simulink model "Trajectory_tracking_full_state_feedback"  (R2023b)
settings: Solver=ode15s  StartTime=0.0  StopTime=tf+ss  FixedStep=Ts/10  MaxStep=Ts  RelTol=1e-12  AbsTol=1e-12
InitFcn:
  | %% Define the points of the curve
  | x=xp;
  | y=yp;
  | 
  | % Number of points
  | n = length(x);
  | 
  | % Initialize the arclength array
  | s = zeros(1, n);
  | 
  | %% Compute the incremental distances and the cumulative sum
  | for i = 2:n
  |     ds = sqrt((x(i) - x(i-1))^2 + (y(i) - y(i-1))^2);
  |     s(i) = s(i-1) + ds;
  | end
  | 
  | s= s/max(s);
  | 
  | [s, unique_indices] = unique(s, 'stable');
  | x = x(unique_indices);
  | y = y(unique_indices);
  | 
  | n = length(x);
  | 
  | %% Compute derivatives with respect to s
  | dx_ds = gradient(x, s);
  | dy_ds = gradient(y, s);
  | 
  | % Compute second derivatives with respect to s
  | d2x_ds2 = gradient(dx_ds, s);
  | d2y_ds2 = gradient(dy_ds, s);
  | 
  | % Compute third derivatives with respect to s
  | d3x_ds3 = gradient(d2x_ds2, s);
  | d3y_ds3 = gradient(d2y_ds2, s);
  | 
  | curvature = sqrt(d2x_ds2.^2+d2y_ds2.^2);
  | 
  | % % Dati Robot
  | CGTF=0.325;
  | CGTR=0.325;
  | Ts = 1/n;
  | 
  | 
  | %% Calcolo path
  | x_s= x;
  | y_s= y;
  | 
  | x_s_prime = dx_ds;
  | y_s_prime = dy_ds;
  | 
  | x_s_second = d2x_ds2;
  | y_s_second = d2y_ds2;
  | 
  | x_s_third = d3x_ds3;
  | y_s_third = d3y_ds3;
  | 
  | v_tilde = sqrt(x_s_prime.^2 + y_s_prime.^2);
  | 
  | theta_s = atan2(y_s_prime./v_tilde,x_s_prime./v_tilde);
  | theta_s_prime = (y_s_second.*x_s_prime-x_s_second.*y_s_prime)./(v_tilde.^2);
  | 
  | phi_s = atan(l*(y_s_second.*x_s_prime-x_s_second.*y_s_prime)./(v_tilde.^3));
  | 
  | w_tilde = (l*v_tilde.*((y_s_third.*x_s_prime-x_s_third.*y_s_prime)-3*(y_s_second.*x_s_prime-x_s_second.*y_s_prime).*(x_s_prime.*x_s_second+y_s_prime.*y_s_second)))./((v_tilde.^6)+(l^2)*(y_s_second.*x_s_prime-x_s_second.*y_s_prime).^2);
  | 
  | %% Time law
  | check=0;
  | t0 = 0;
  | tf = 1;
  | K=1;
  | while (~check)
  | 
  |     a0 = s(:,1);
  |     a1 = 0;
  |     a2 = 3/(tf^2)*(s(:,n)-s(:,1));
  |     a3 = -2/(tf^3)*(s(:,n)-s(:,1));
  | 
  |     % % Define the boundary conditions for s(t)
  |     % t0 = 0; % initial time
  |     % t_end = tf; % end time
  |     % s0 = s(:,1); % initial arc length
  |     % s_end = s(:,n); % end arc length
  |     % v0 = 0; % initial velocity
  |     % v_end = 0; % end velocity
  |     % a0 = 0; % initial acceleration
  |     % a_end = 0; % end acceleration
  |     %
  |     % % Set up the system of equations for quintic polynomial
  |     % A = [
  |     %     1, t0, t0^2, t0^3, t0^4, t0^5;
  |     %     1, t_end, t_end^2, t_end^3, t_end^4, t_end^5;
  |     %     0, 1, 2*t0, 3*t0^2, 4*t0^3, 5*t0^4;
  |     %     0, 1, 2*t_end, 3*t_end^2, 4*t_end^3, 5*t_end^4;
  |     %     0, 0, 2, 6*t0, 12*t0^2, 20*t0^3;
  |     %     0, 0, 2, 6*t_end, 12*t_end^2, 20*t_end^3
  |     % ];
  |     %
  |     % b = [s0; s_end; v0; v_end; a0; a_end];
  |     %
  |     % % Solve for the coefficients
  |     % coefficients = A\b;
  |     %
  |     % % Extract the coefficients
  |     % a0 = coefficients(1);
  |     % a1 = coefficients(2);
  |     % a2 = coefficients(3);
  |     % a3 = coefficients(4);
  |     % a4 = coefficients(5);
  |     % a5 = coefficients(6);
  | 
  |     % Define the quintic polynomial function s(t)
  |     % s_t = @(t) a0 + a1*t + a2*t^2 + a3*t^3 + a4*t^4 + a5*t^5;
  |     s_t = @(t) a3*t^3 + a2*t^2 + a1*t + a0;
  | 
  |     % Create x(t) and y(t)
  |     x_t = @(t) interp1(s, x_s, s_t(t),'spline','extrap');
  |     y_t = @(t) interp1(s, y_s, s_t(t),'spline','extrap');
  | 
  |     t_values = linspace(0, tf, n);
  | 
  |     x_values = arrayfun(@(t) x_t(t),t_values);
  |     y_values = arrayfun(@(t) y_t(t),t_values);
  | 
  |     s_t_dot = 3*a3*t_values.^2 + 2*a2*t_values + a1;
  |     % s_t_dot = a1 + 2*a2*t_values + 3*a3*t_values.^2 + 4*a4*t_values.^3 + 5*a5*t_values.^4;
  | 
  |     x_t_dot = x_s_prime.*s_t_dot;
  |     y_t_dot = y_s_prime.*s_t_dot;
  | 
  |     v_t = v_tilde.*s_t_dot;
  | 
  |     w_t = w_tilde.*s_t_dot;
  | 
  |     theta_t = @(t) interp1(s, theta_s, s_t(t),'spline','extrap');
  |     theta_values = arrayfun(@(t) theta_t(t),t_values);
  | 
  |     theta_t_dot = theta_s_prime.*s_t_dot;
  | 
  |     phi_t = @(t) interp1(s, phi_s, s_t(t),'spline','extrap');
  |     phi_values = arrayfun(@(t) phi_t(t),t_values);
  | 
  |     theta_t_dot_lim = tan(phi_lim)/l*vlim;
  | 
  |     v_max = max(abs(v_t));
  |     w_max = max(abs(w_t));
  |     theta_max = max(abs(theta_t_dot));
  |     phi_max = max(abs(phi_values));
  | 
  |     check = 1;
  | 
  |     if ((v_max>vlim || w_max>wlim || theta_max>theta_t_dot_lim)) %&& phi_max<phi_lim )
  |         Kmax = [v_max/vlim w_max/wlim theta_max/theta_t_dot_lim ];
  |         K = max(Kmax);
  |         tf = tf*K;
  |         check=0;
  |     end
  | 
  | end
  | 
  | 
  | v_t_reference = timeseries(v_t,t_values);
  | w_t_reference = timeseries(w_t,t_values);
  | theta_t_reference = timeseries(theta_values,t_values);
  | theta_t_dot_reference = timeseries(theta_t_dot,t_values);
  | phi_t_reference = timeseries(phi_values,t_values);
  | 
  | x_t_reference = timeseries(x_values,t_values);
  | y_t_reference = timeseries(y_values,t_values);
  | x_dot_t_reference = timeseries(x_t_dot,t_values);
  | y_dot_t_reference = timeseries(y_t_dot,t_values);
undefined symbols (not defined in the file): b, k1, k2, l, phi_lim, vlim, wlim
settings Model: Creator=avvmi  LastModifiedBy=avvmi
settings DebuggingCC: UnderSpecifiedDimensionMsg=error

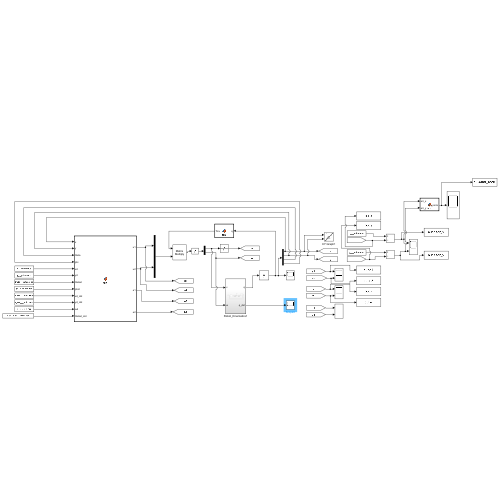
[thumbnail: Simulink's stored preview of the top-level diagram]
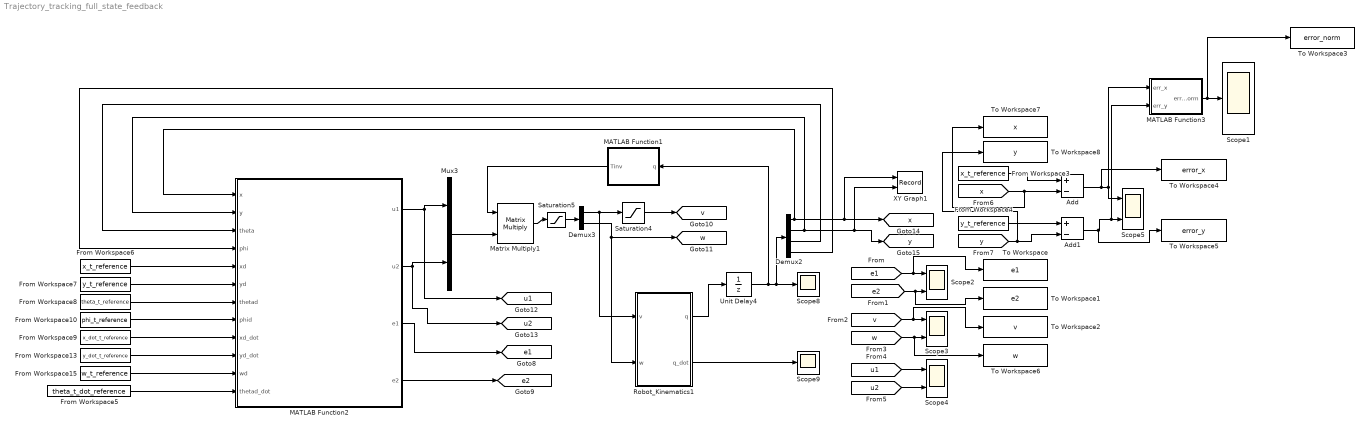
== system Trajectory_tracking_full_state_feedback ==
  Add : Sum  Inputs=+-
  Add1 : Sum  Inputs=+-
  Demux2 : Demux
  Demux3 : Demux  Outputs=2
  From Workspace10 : FromWorkspace  VariableName=phi_t_reference  OutDataTypeStr=double  SampleTime=Ts  OutputAfterFinalValue=Holding final value
  From Workspace13 : FromWorkspace  VariableName=y_dot_t_reference  OutDataTypeStr=double  SampleTime=Ts  OutputAfterFinalValue=Holding final value
  From Workspace15 : FromWorkspace  VariableName=w_t_reference  OutDataTypeStr=double  SampleTime=Ts  OutputAfterFinalValue=Holding final value
  From Workspace3 : FromWorkspace  VariableName=x_t_reference  SampleTime=Ts  OutputAfterFinalValue=Holding final value
  From Workspace4 : FromWorkspace  VariableName=y_t_reference  SampleTime=Ts  OutputAfterFinalValue=Holding final value
  From Workspace5 : FromWorkspace  VariableName=theta_t_dot_reference  OutDataTypeStr=double  SampleTime=Ts  OutputAfterFinalValue=Holding final value
  From Workspace6 : FromWorkspace  VariableName=x_t_reference  OutDataTypeStr=double  SampleTime=Ts  OutputAfterFinalValue=Holding final value
  From Workspace7 : FromWorkspace  VariableName=y_t_reference  OutDataTypeStr=double  SampleTime=Ts  OutputAfterFinalValue=Holding final value
  From Workspace8 : FromWorkspace  VariableName=theta_t_reference  OutDataTypeStr=double  SampleTime=Ts  OutputAfterFinalValue=Holding final value
  From Workspace9 : FromWorkspace  VariableName=x_dot_t_reference  OutDataTypeStr=double  SampleTime=Ts  OutputAfterFinalValue=Holding final value
  MATLAB Function1 : MATLAB Function  TreatAsAtomicUnit=on
  MATLAB Function2 : MATLAB Function  TreatAsAtomicUnit=on
  MATLAB Function3 : MATLAB Function  TreatAsAtomicUnit=on
  Matrix Multiply1 : Product  Multiplication=Matrix(*)
  Mux3 : Mux  Inputs=2
  Robot_Kinematics1 : Subsystem
  Saturation4 : Saturate  UpperLimit=inf  LowerLimit=0
  Saturation5 : Saturate  UpperLimit=[vlim wlim]'  LowerLimit=-[vlim wlim]'
  Scope1 : Scope
  Scope{2..5} (4 alike) : Scope  NumInputPorts=2
  Scope8 : Scope
  Scope9 : Scope
  To Workspace : ToWorkspace  VariableName=e1  SaveFormat=Timeseries  SampleTime=-1
  To Workspace1 : ToWorkspace  VariableName=e2  SaveFormat=Timeseries  SampleTime=-1
  To Workspace2 : ToWorkspace  VariableName=v  SaveFormat=Timeseries  SampleTime=-1
  To Workspace3 : ToWorkspace  VariableName=error_norm  SaveFormat=Timeseries  SampleTime=-1
  To Workspace4 : ToWorkspace  VariableName=error_x  SaveFormat=Timeseries  SampleTime=-1
  To Workspace5 : ToWorkspace  VariableName=error_y  SaveFormat=Timeseries  SampleTime=-1
  To Workspace6 : ToWorkspace  VariableName=w  SaveFormat=Timeseries  SampleTime=-1
  To Workspace7 : ToWorkspace  VariableName=x  SaveFormat=Timeseries  SampleTime=-1
  To Workspace8 : ToWorkspace  VariableName=y  SaveFormat=Timeseries  SampleTime=-1
  Unit Delay4 : UnitDelay  InitialCondition=[x_values(:,1) y_values(:,1) theta_values(:,1) phi_values(:,1)]'  SampleTime=Ts  HasFrameUpgradeWarning=on
  XY Graph1 : Record  FileSettingsInternal="{\"entries\":[{\"content\":{\"excelSettings\":{\"content\":{},\"type\":\"Streamout.ExcelSettings\"}},\"type\":\"Streamout.FileSettingStorage\",\"uuid\":\"\"}],\"packageUris\":[\"http:\\/\\/schema.mathworks.com\\/mf0\\/streamout_blocks\\/R2020a\"],\"version\":\"1.0\"}"  Layout=[1 1]  SignalsInternal="{\"entries\":[{\"content\":{\"signals\":[{\"content\":{\"blockPath\":[],\"dimensions\":[1],\"domain\":\"\",\"lineColor\":\"#ff6929\",\"plots\":[1],\"port\":1,\"sid\":[\"\"],\"signalID\":19,\"signalName\":\"Demux2:1\"},\"type\":\"RecordBlkView.Signal\",\"uuid\":\"\"},{\"content\":{\"blockPath\":[],\"dimensions\":[1],\"domain\":\"\",\"lineColor\":\"#b746ff\",\"plots\":[1],\"port\":2,\"sid\":[\"\"],\"signalID\":23,\"signalName\":\"Demux2:2\"},\"type\":\"RecordBlkView.Signal\",\"uuid\":\"\"}]},\"type\":\"RecordBlkView.InputSignals\",\"uuid\":\"\"}],\"packageUris\":[\"http:\\/\\/schema.mathworks.com\\/mf0\\/streamout_blocks\\/R2020a\"],\"version\":\"1.0\"}"  VisualizationBindings="{\"xyplotplugin\":{\"info\":[{\"series\":[{\"bindingParametersList\":[{\"parameter\":\"X-Axis\",\"signalID\":19,\"signalName\":\"Demux2:1\"},{\"parameter\":\"Y-Axis\",\"signalID\":23,\"signalName\":\"Demux2:2\"}],\"seriesID\":4500}],\"subplotID\":1}]}}"  CompatibilityTag=XY
  tag scope: e1=global, e2=global, u1=global, u2=global, v=global, w=global, x=global, y=global
  wires:
  [e2] -> To Workspace1/1, Scope2/2
  [v] -> To Workspace2/1, Scope3/1
  [w] -> To Workspace6/1, Scope3/2
  [u1] -> Scope4/1
  [u2] -> Scope4/2
  [x] -> To Workspace7/1, Add/2
  [y] -> To Workspace8/1, Add1/2
  From Workspace3/1 -> Add/1
  From Workspace4/1 -> Add1/1
  MATLAB Function2/3(e1) -> [e1]
  Saturation5/1 -> Demux3/1
  From Workspace8/1 -> MATLAB Function2/7(thetad)
  Demux2/4 -> MATLAB Function2/4(phi)
  From Workspace5/1 -> MATLAB Function2/12(thetad_dot)
  Matrix Multiply1/1 -> Saturation5/1
  From Workspace13/1 -> MATLAB Function2/10(yd_dot)
  Demux2/2 -> MATLAB Function2/2(y), [y], XY Graph1/2
  Saturation4/1 -> [v]
  MATLAB Function2/1(u1) -> Mux3/1, [u1]
  MATLAB Function2/2(u2) -> Mux3/2, [u2]
  Demux2/1 -> MATLAB Function2/1(x), [x], XY Graph1/1
  From Workspace6/1 -> MATLAB Function2/5(xd)
  Demux3/1 -> Robot_Kinematics1/1(v), Saturation4/1
  Mux3/1 -> Matrix Multiply1/2
  From Workspace10/1 -> MATLAB Function2/8(phid)
  From Workspace9/1 -> MATLAB Function2/9(xd_dot)
  Demux3/2 -> Robot_Kinematics1/2(w), [w]
  From Workspace7/1 -> MATLAB Function2/6(yd)
  Robot_Kinematics1/2(q_dot) -> Scope9/1
  MATLAB Function2/4(e2) -> [e2]
  From Workspace15/1 -> MATLAB Function2/11(wd)
  MATLAB Function1/1(Tinv) -> Matrix Multiply1/1
  Demux2/3 -> MATLAB Function2/3(theta)
  Robot_Kinematics1/1(q) -> Unit Delay4/1
  Unit Delay4/1 -> MATLAB Function1/1(q), Demux2/1, Scope8/1
  [e1] -> To Workspace/1, Scope2/1
  Add/1 -> To Workspace4/1, Scope5/1, MATLAB Function3/1(err_x)
  MATLAB Function3/1(err_norm) -> To Workspace3/1, Scope1/1
  Add1/1 -> To Workspace5/1, MATLAB Function3/2(err_y), Scope5/2

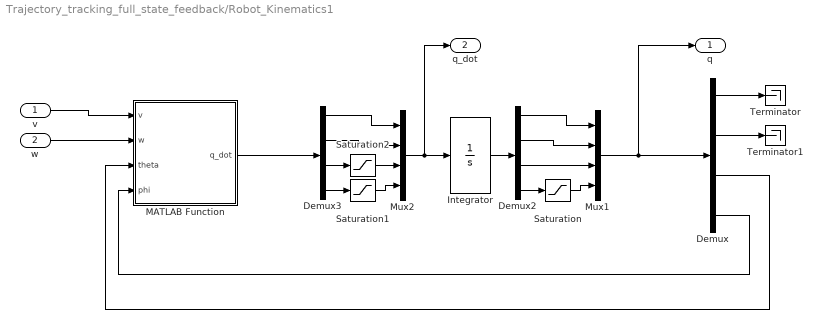
== system Trajectory_tracking_full_state_feedback/Robot_Kinematics1 ==
  v : Inport
  w : Inport  Port=2
  Demux : Demux
  Demux2 : Demux
  Demux3 : Demux
  Integrator : Integrator  InitialCondition=[x_values(:,1) y_values(:,1) theta_values(:,1) phi_values(:,1)]'  UpperSaturationLimit=[inf inf inf 1.5]'  LowerSaturationLimit=[-inf -inf -inf -1.5]'
  MATLAB Function : MATLAB Function  TreatAsAtomicUnit=on
  Mux1 : Mux
  Mux2 : Mux
  Saturation : Saturate  UpperLimit=phi_lim  LowerLimit=-phi_lim
  Saturation1 : Saturate  UpperLimit=wlim  LowerLimit=-wlim
  Saturation2 : Saturate  UpperLimit=theta_t_dot_lim  LowerLimit=-theta_t_dot_lim
  Terminator : Terminator
  Terminator1 : Terminator
  q : Outport
  q_dot : Outport  Port=2
  wires:
  Integrator/1 -> Demux2/1
  Demux/3 -> MATLAB Function/3(theta)
  Demux/4 -> MATLAB Function/4(phi)
  v/1 -> MATLAB Function/1(v)
  w/1 -> MATLAB Function/2(w)
  Demux/1 -> Terminator/1
  Demux/2 -> Terminator1/1
  Demux2/4 -> Saturation/1
  Mux1/1 -> q/1, Demux/1
  Saturation/1 -> Mux1/4
  Demux2/3 -> Mux1/3
  Demux2/2 -> Mux1/2
  Demux2/1 -> Mux1/1
  Saturation1/1 -> Mux2/4
  Demux3/2 -> Mux2/2
  Demux3/4 -> Saturation1/1
  Demux3/3 -> Saturation2/1
  MATLAB Function/1(q_dot) -> Demux3/1
  Demux3/1 -> Mux2/1
  Mux2/1 -> q_dot/1, Integrator/1
  Saturation2/1 -> Mux2/3

== matlab function Trajectory_tracking_full_state_feedback/MATLAB Function3 ==
  data: err_x input; err_norm output; err_y input
function err_norm = fcn(err_x,err_y)


err_norm = sqrt((err_x^2)+(err_y^2));

== matlab function Trajectory_tracking_full_state_feedback/MATLAB Function1 ==
  data: q input; Tinv output; b parameter; l parameter
function Tinv = fcn(q,b,l)

T = [cos(q(3))-tan(q(4))*sin(q(3))-(b/l)*tan(q(4))*sin(q(3)+q(4)) -b*sin(q(3)+q(4));
    sin(q(3))+tan(q(4))*cos(q(3))+(b/l)*tan(q(4))*cos(q(3)+q(4)) b*cos(q(3)+q(4))];

Tinv= inv(T);

== matlab function Trajectory_tracking_full_state_feedback/MATLAB Function2 ==
  data: x input; u1 output; u2 output; y input; theta input; phi input; xd input; yd input; thetad input; phid input; xd_dot input; yd_dot input; wd input; thetad_dot input; e1 output; e2 output; b parameter; l parameter; Ts parameter; d2x_ds2 parameter; d2y_ds2 parameter; k1 parameter; k2 parameter
function [u1,u2,e1,e2]=fcn(x,y,theta,phi,xd,yd,thetad,phid,xd_dot,yd_dot,wd,thetad_dot,b,l,Ts,d2x_ds2, d2y_ds2,k1, k2)

persistent sum1;
persistent sum2;

if isempty(sum1) || isempty(sum2) 
         sum1 = 0;
         sum2 = 0;
end


e1 = (xd+l*cos(thetad)+b*cos(thetad+phid))-(x+l*cos(theta)+b*cos(theta+phi));
e2 = (yd+l*sin(thetad)+b*sin(thetad+phid))-(y+l*sin(theta)+b*sin(theta+phi));

% sum1=sum1+e1*Ts;
% sum2=sum2+e2*Ts;
% k1=3;
% k2=k1*(max(d2y_ds2)/max(d2x_ds2));
% k3=0;
% k4=0;

u1 = xd_dot-l*thetad_dot*sin(thetad)-b*(thetad_dot+wd)*sin(thetad+phid) + k1*e1; 
u2 = yd_dot+l*thetad_dot*cos(thetad)+b*(thetad_dot+wd)*cos(thetad+phid) + k2*e2;

== matlab function Trajectory_tracking_full_state_feedback/Robot_Kinematics1/MATLAB Function ==
  data: v input; q_dot output; w input; theta input; phi input; l parameter
function q_dot = fcn(v,w,theta,phi,l)

x_dot = cos(theta)*v;
y_dot = sin(theta)*v;
theta_dot = (tan(phi)/l)*v;
phi_dot = w;

q_dot = [x_dot y_dot theta_dot phi_dot]';
